simulink subsystem "Pump_step_algortihm"  (R2022b)
settings: Solver=VariableStepAuto  StartTime=0.0  StopTime=inf  RelTol=1e-3
model mask{start_frequncy=63}
  mask prompts: start_frequncy "Start frequncy [0-100]"
settings Model: DefaultTestHarness=Pump_step_algortihm_Harness1  Creator=pppc  LastModifiedBy=pppc

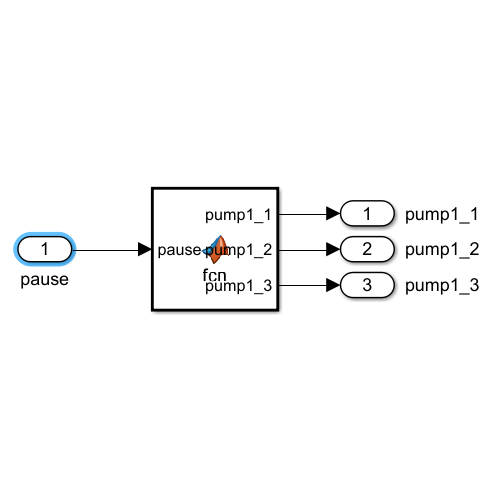
[thumbnail: Simulink's stored preview of the top-level diagram]
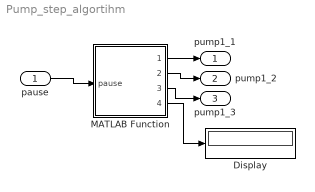
== system Pump_step_algortihm ==
  pause : Inport
  Display : Display
  MATLAB Function : MATLAB Function  TreatAsAtomicUnit=on  SystemSampleTime=1
  pump1_1 : Outport
  pump1_2 : Outport  Port=2
  pump1_3 : Outport  Port=3
  wires:
  MATLAB Function/2(pump1_2) -> pump1_2/1
  MATLAB Function/3(pump1_3) -> pump1_3/1
  MATLAB Function/1(pump1_1) -> pump1_1/1
  pause/1 -> MATLAB Function/1(pause)
  MATLAB Function/4(time_out) -> Display/1

== matlab function Pump_step_algortihm/MATLAB Function ==
  data: pause input; pump1_1 output; pump1_2 output; pump1_3 output; start_frequncy parameter; time_out output
function [pump1_1, pump1_2, pump1_3, time_out]  = fcn(pause,start_frequncy)
persistent time;
if(isempty(time)); time = 0; end
persistent n_pumps;
if(isempty(n_pumps)); n_pumps = 1;  end
persistent frequncy;
if(isempty(frequncy)); frequncy = start_frequncy;  end

pump1_1 = 0;
pump1_2 = 0;
pump1_3 = 0;
time_out = time;

if(pause>0)
   time = -180;
   disp("Pausing due to high pause signal");
   return
end

time = time + 1;
if(time > 59)
    time = 0 ;
    frequncy = frequncy + 4;
    if(frequncy>99)
        frequncy = start_frequncy;
        n_pumps  = n_pumps + 1;
    end 
end

switch n_pumps
    case 1
        pump1_1 = frequncy;
    case 2
        pump1_1 = frequncy;
        pump1_2 = frequncy;
    case 3
        pump1_1 = frequncy;
        pump1_2 = frequncy;
        pump1_3 = frequncy;
end
